simulink model "Program_1_SIR_Italy_R2018b 2"  (R2018b)
settings: Solver=FixedStepAuto  StartTime=0.0  StopTime=180  FixedStep=0.001  RelTol=1e-9  AbsTol=1e-9
values from neighbouring files (symbols this model uses):
  a = 0.5    [Main_SIR_Italy_Program_1 2.m]
  beta = 1.53602767817435    (= 1.53602767817)    [Main_SIR_Italy_Program_1 2.m]
  gamma1 = 0.0128250346772537    (= 0.0128250346773)    [Main_SIR_Italy_Program_1 2.m]
  gamma2 = 0.00483679113978549    (= 0.00483679113979)    [Main_SIR_Italy_Program_1 2.m]
  gamma3 = 0.149311333504727    (= 0.149311333505)    [Main_SIR_Italy_Program_1 2.m]
  I0 = 1    [Main_SIR_Italy_Program_1 2.m]
  P = 60*10^6    (= 60000000)    [Main_SIR_Italy_Program_1 2.m]
  R0 = 0    [Main_SIR_Italy_Program_1 2.m]
  zeta1 = -2.03011707682403    (= -2.03011707682)    [Main_SIR_Italy_Program_1 2.m]
  zeta2 = -2.60970797840359    (= -2.6097079784)    [Main_SIR_Italy_Program_1 2.m]
  zeta3 = -2.55914577598691    (= -2.55914577599)    [Main_SIR_Italy_Program_1 2.m]
libraries: fuzblock x3
settings Model: OrderedModelArguments=off  Creator=ismae  LastModifiedBy=ismae
settings SolverCC: SolverResetMethod=Robust
settings DataIOCC: ReturnWorkspaceOutputs=on

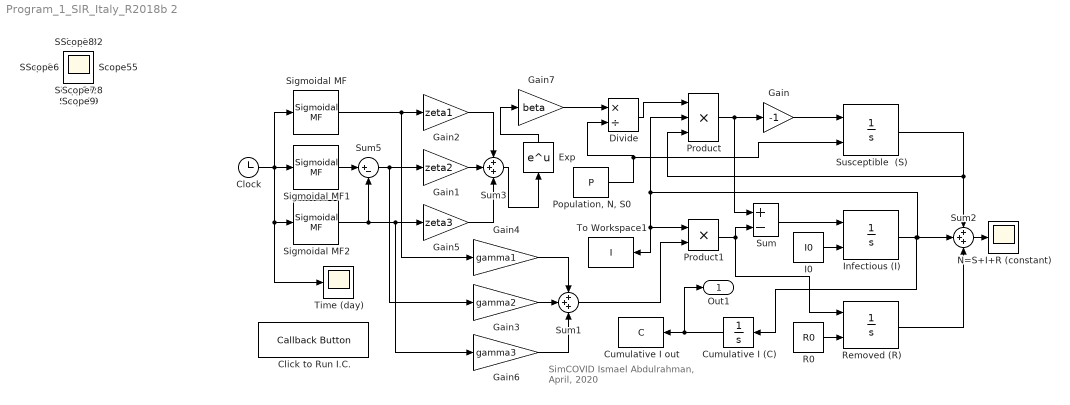
== system Program_1_SIR_Italy_R2018b 2 ==
  note: SimCOVID
      | Ismael Abdulrahman, April, 2020
  Click to Run I.C. : CallbackButton  Description=Run this callback button first to evaluate the initial values for the parameters  WebBlockId=264
      settings: ClickFcn=|
      | P   = 60*10^6; % Population, Susceptible, N, S0
      | I0  = 1;       % Initial value for "Infectious"
      | R0  = 0;       % Initial value for "Removed"
      | st1 = 40;      % starting time 1 (step time)
      | st2 = 52;      % starting time 2 (step time)
      | %==========================================================================
      | a=0.5;
      | gamma=0.05;
      | beta    = 1.53602767817435;
      | gamma1  =  0.0128250346772537;
      | gamma2  = 0.00483679113978549;
      | gamma3  = 0.149311333504727;
      | zeta1   = -2.03011707682403;
      | zeta2   = -2.60970797840359;
      | zeta3   = -2.55914577598691;
      | I1 = xlsread('COVID-19-geographic-disbtribution-worldwide-2020-04-07','Italy','E:E');
      | Im  = flip(I1);  Im=Im(32:end); %  The first 31 elements are zeros
      | Cm  =cumsum(Im);            x   % Cumulative sum of I
      | t  = 1:length(Cm);
      | xy = [t' Cm];
      | xy0 = [t' Im];
  Clock : Clock
  Cumulative I (C) : Integrator
  Cumulative I out : ToWorkspace  VariableName=C  SampleTime=-1
      settings: Save2DSignal=2-D array (concatenate along first dimension)
  Divide : Product  Inputs=*/
  Exp : Math  SaturateOnIntegerOverflow=on
  Gain : Gain  Gain=-1
  Gain1 : Gain  Gain=zeta2
  Gain2 : Gain  Gain=zeta1
  Gain3 : Gain  Gain=gamma2
  Gain4 : Gain  Gain=gamma1
  Gain5 : Gain  Gain=zeta3
  Gain6 : Gain  Gain=gamma3
  Gain7 : Gain  Gain=beta
  I0 : Constant  Value=I0
  Infectious (I) : Integrator  InitialConditionSource=external
  N=S+I+R (constant) : Scope
  "Population, N, S0" : Constant  Value=P
  Product : Product  Inputs=3
  Product1 : Product
  R0 : Constant  Value=R0
  Removed (R) : Integrator  InitialConditionSource=external
  Sigmoidal MF : fuzblock/Membership  Functions/Sigmoidal MF  a=-a  c=st1
      settings: SourceProductName=Fuzzy Logic Toolbox  SourceProductBaseCode=FL
  Sigmoidal MF1 : fuzblock/Membership  Functions/Sigmoidal MF  a=a  c=st1
      settings: SourceProductName=Fuzzy Logic Toolbox  SourceProductBaseCode=FL
  Sigmoidal MF2 : fuzblock/Membership  Functions/Sigmoidal MF  a=a  c=st2
      settings: SourceProductName=Fuzzy Logic Toolbox  SourceProductBaseCode=FL
  Sum : Sum  Inputs=+-
  Sum1 : Sum  Inputs=+++
  Sum2 : Sum  Inputs=+++
  Sum3 : Sum  Inputs=+++
  Sum5 : Sum  Inputs=|+-
  Susceptible  (S) : Integrator  InitialConditionSource=external  InitialCondition=10000
  Time (day) : Scope
  To Workspace1 : ToWorkspace  VariableName=I  SampleTime=-1
      settings: Save2DSignal=2-D array (concatenate along first dimension)
  Out1 : Outport
  Scope{,1..32} (33 alike) : Scope
  wires:
  Product/1 -> Gain/1, Sum/1
  Divide/1 -> Product/1
  Sum/1 -> Infectious (I)/1
  I0/1 -> Infectious (I)/2
  "Population, N, S0"/1 -> Susceptible  (S)/2, Divide/2
  Sum2/1 -> N=S+I+R (constant)/1
  R0/1 -> Removed (R)/2
  Product1/1 -> Removed (R)/1, Sum/2
  Gain5/1 -> Sum3/3
  Gain1/1 -> Sum3/2
  Gain2/1 -> Sum3/1
  Susceptible  (S)/1 -> Product/3, Sum2/1
  Gain/1 -> Susceptible  (S)/1
  Infectious (I)/1 -> Product1/1, To Workspace1/1, Product/2, Sum2/2, Cumulative I (C)/1
  Removed (R)/1 -> Sum2/3
  Cumulative I (C)/1 -> Cumulative I out/1, Out1/1
  Sum3/1 -> Exp/1
  Exp/1 -> Gain7/1
  Sum1/1 -> Product1/2
  Sigmoidal MF/1 -> Gain4/1, Gain2/1
  Sigmoidal MF1/1 -> Sum5/1
  Gain4/1 -> Sum1/1
  Sigmoidal MF2/1 -> Gain6/1, Gain5/1, Sum5/2
  Sum5/1 -> Gain3/1, Gain1/1
  Gain7/1 -> Divide/1
  Gain6/1 -> Sum1/3
  Gain3/1 -> Sum1/2
  Clock/1 -> Sigmoidal MF/1, Sigmoidal MF1/1, Sigmoidal MF2/1, Time (day)/1
